simulink model "tpi2series"  (R2017b)
settings: Solver=VariableStepAuto  StartTime=0.0  StopTime=3  MaxStep=1e-4  RelTol=1e-3
values from neighbouring files (symbols this model uses):
  fdclinkcap = 100e-6    (= 0.0001)    [tpi2parallelrunner.m]    (also in tpi2seriesrunner.m = 0.01; tpireloadedrunner.m = 0.01)
  fdclinkres = 1e-6    (= 1e-06)    [tpi2parallelrunner.m]    (also in tpi2seriesrunner.m; tpireloadedrunner.m)
  fma = 0.9    [tpi2parallelrunner.m]    (also in tpi2seriesrunner.m; tpireloadedrunner.m)
  fswfreq = 20000    [tpi2parallelrunner.m]    (also in tpi2seriesrunner.m = 2050; tpireloadedrunner.m)
  Rin = 1    [tpi2parallelrunner.m]    (also in tpi2seriesrunner.m = 1e-16; tpireloadedrunner.m)
  sdclinkcap = 1e-2    (= 0.01)    [tpi2seriesrunner.m]    (also in tpireloadedrunner.m)
  sdclinkres = 1e-6    (= 1e-06)    [tpi2seriesrunner.m]    (also in tpireloadedrunner.m)
  sma = 0.9    [tpi2parallelrunner.m]    (also in tpi2seriesrunner.m; tpireloadedrunner.m)
  sswfreq = 20000    [tpi2parallelrunner.m]    (also in tpi2seriesrunner.m = 2050; tpireloadedrunner.m)
undefined symbols (not defined in the file or in its folder): fdcin, fdclink1cap
libraries: powerlib x22, simulink x6, powerlib_meascontrol x2
settings Model: Creator=Orhun  LastModifiedBy=Orhun

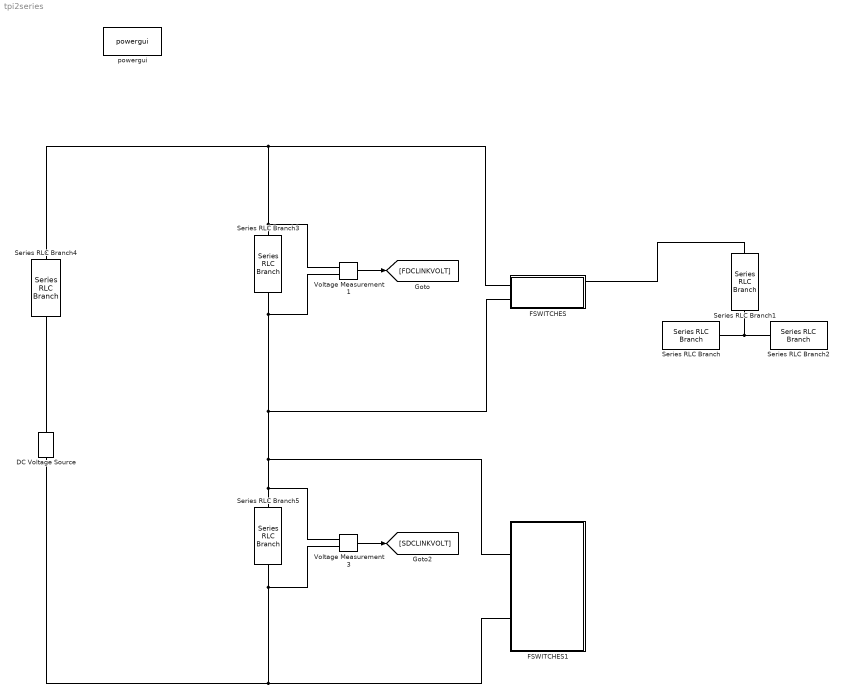
== system tpi2series ==
  DC Voltage Source : powerlib/Electrical Sources/DC Voltage Source  Amplitude=fdcin  Measurements=None
  FSWITCHES : Subsystem
  FSWITCHES1 : Subsystem
  Series RLC Branch : powerlib/Elements/Series RLC Branch  LConnTagsString=__new0  RConnTagsString=__new0  BranchType=RL  Resistance=5  Inductance=2e-3  SetiL0=off  InitialCurrent=0  Capacitance=0  Setx0=off  InitialVoltage=0  Measurements=None
  Series RLC Branch1 : powerlib/Elements/Series RLC Branch  LConnTagsString=__new0  RConnTagsString=__new0  BranchType=RL  Resistance=5  Inductance=2e-3  SetiL0=off  InitialCurrent=0  Capacitance=0  Setx0=off  InitialVoltage=0  Measurements=None
  Series RLC Branch2 : powerlib/Elements/Series RLC Branch  LConnTagsString=__new0  RConnTagsString=__new0  BranchType=RL  Resistance=5  Inductance=2e-3  SetiL0=off  InitialCurrent=0  Capacitance=0  Setx0=off  InitialVoltage=0  Measurements=None
  Series RLC Branch3 : powerlib/Elements/Series RLC Branch  LConnTagsString=__new0  RConnTagsString=__new0  BranchType=RC  Resistance=fdclinkres  Inductance=0  SetiL0=off  InitialCurrent=0  Capacitance=fdclinkcap  Setx0=off  InitialVoltage=0  Measurements=None
  Series RLC Branch4 : powerlib/Elements/Series RLC Branch  LConnTagsString=__new0  RConnTagsString=__new0  BranchType=R  Resistance=Rin  Inductance=0  SetiL0=off  InitialCurrent=0  Capacitance=fdclink1cap  Setx0=off  InitialVoltage=0  Measurements=None
  Series RLC Branch5 : powerlib/Elements/Series RLC Branch  LConnTagsString=__new0  RConnTagsString=__new0  BranchType=RC  Resistance=sdclinkres  Inductance=0  SetiL0=off  InitialCurrent=0  Capacitance=sdclinkcap  Setx0=off  InitialVoltage=0  Measurements=None
  Voltage Measurement1 : powerlib/Measurements/Voltage Measurement  PhasorSimulation=off  OutputType=Complex  PSBequivalent=0
  Voltage Measurement3 : powerlib/Measurements/Voltage Measurement  PhasorSimulation=off  OutputType=Complex  PSBequivalent=0
  powergui : powerlib/powergui  Priority=1  SimulationMode=Continuous  SampleTime=50e-6  frequency=60  Iterations=50  frequencyindice=0  Pbase=100e6  ErrMax=1e-4  UnitsV=kV  UnitsW=MW  buscounter=0  FunctionMessages=off  echomessages=off  EnableUseOfTLC=off  CurrentSourceSwitches=off  DisableSnubberDevices=off  DisableRonSwitches=off  DisableVfSwitches=off  DisplayEquations=off  SolverType=Tustin/Backward Euler (TBE)  Interpol=off  ExternalGateDelay=off  methode=off  Ts=100  x0status=blocks  SPID=on  SwTol=0  HookPort=off  RestoreLinks=warning  ResistiveCurrentMeasurement=off  Frange=[0:2:500]  Ylog=off  Xlog=on  ShowGrid=off  save=off  variable=ZData  structure=0  ZoomFFT=off  StartTime=0.0  cycles=1  DisplayStyle=1  fundamental=60  FreqAxis=off  MaxFrequency=1000  frequencyindicesteady=1  RmsSteady=1  display=off
  wires:
  Voltage Measurement1/1 -> [FDCLINKVOLT]
  Voltage Measurement3/1 -> [SDCLINKVOLT]
  connections:
  Series RLC Branch2/RConn1 -- Series RLC Branch1/LConn1 -- Series RLC Branch/LConn1
  Series RLC Branch3/LConn1 -- Series RLC Branch4/LConn1 -- FSWITCHES/LConn1 -- Voltage Measurement1/LConn1
  Voltage Measurement1/LConn2 -- FSWITCHES1/LConn1 -- Voltage Measurement3/LConn1 -- Series RLC Branch5/LConn1 -- FSWITCHES/LConn2 -- Series RLC Branch3/RConn1
  Series RLC Branch4/RConn1 -- DC Voltage Source/RConn1
  Voltage Measurement3/LConn2 -- DC Voltage Source/LConn1 -- FSWITCHES1/LConn2 -- Series RLC Branch5/RConn1
  FSWITCHES/RConn1 -- Series RLC Branch1/RConn1

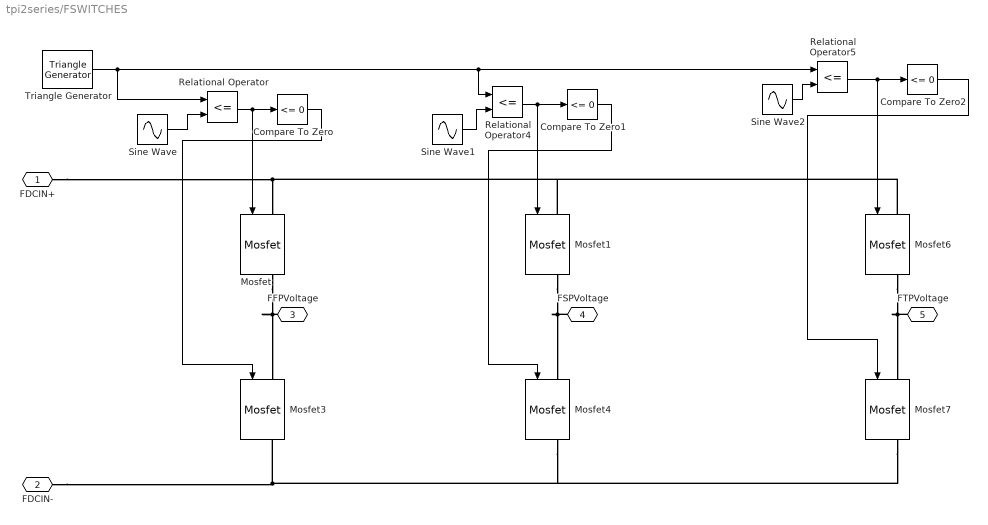
== system tpi2series/FSWITCHES ==
  Compare To Zero : simulink/Logic and Bit Operations/Compare To Zero  relop=<=  OutDataTypeStr=boolean
  Compare To Zero1 : simulink/Logic and Bit Operations/Compare To Zero  relop=<=  OutDataTypeStr=boolean
  Compare To Zero2 : simulink/Logic and Bit Operations/Compare To Zero  relop=<=  OutDataTypeStr=boolean
  Mosfet{,1,3..4,6..7} (6 alike) : powerlib/Power Electronics/Mosfet  Ron=2e-3  Lon=0  Rd=0.01  Vfd=0  IC=0  Rs=1e5  Cs=inf  Measurements=on
  Relational Operator : RelationalOperator  Operator=<=  OutDataTypeStr=boolean  RndMeth=Simplest
  Relational Operator4 : RelationalOperator  Operator=<=  OutDataTypeStr=boolean  RndMeth=Simplest
  Relational Operator5 : RelationalOperator  Operator=<=  OutDataTypeStr=boolean  RndMeth=Simplest
  Sine Wave : Sin  Amplitude=fma  Frequency=2*pi*fswfreq  SampleTime=0
  Sine Wave1 : Sin  Amplitude=fma  Frequency=2*pi*fswfreq  Phase=2*pi/3  SampleTime=0
  Sine Wave2 : Sin  Amplitude=fma  Frequency=2*pi*fswfreq  Phase=4*pi/3  SampleTime=0
  Triangle Generator : powerlib_meascontrol/Pulse & Signal Generators/Triangle Generator  Freq=fswfreq  Phase=90  Ts=0
  FDCIN+ : PMIOPort  Port=1  Side=Left
  FDCIN- : PMIOPort  Port=2  Side=Left
  FFPVoltage : PMIOPort  Port=3  Side=Right
  FSPVoltage : PMIOPort  Port=4  Side=Right
  FTPVoltage : PMIOPort  Port=5  Side=Right
  wires:
  Sine Wave/1 -> Relational Operator/2
  Triangle Generator/1 -> Relational Operator5/1, Relational Operator4/1, Relational Operator/1
  Relational Operator4/1 -> Mosfet1/1, Compare To Zero1/1
  Sine Wave2/1 -> Relational Operator5/2
  Sine Wave1/1 -> Relational Operator4/2
  Relational Operator/1 -> Compare To Zero/1, Mosfet/1
  Compare To Zero/1 -> Mosfet3/1
  Compare To Zero1/1 -> Mosfet4/1
  Compare To Zero2/1 -> Mosfet7/1
  Relational Operator5/1 -> Mosfet6/1, Compare To Zero2/1
  connections:
  Mosfet6/RConn1 -- FTPVoltage/RConn1 -- Mosfet7/LConn1
  Mosfet/RConn1 -- FFPVoltage/RConn1 -- Mosfet3/LConn1
  Mosfet1/RConn1 -- FSPVoltage/RConn1 -- Mosfet4/LConn1
  FDCIN+/RConn1 -- Mosfet6/LConn1 -- Mosfet1/LConn1 -- Mosfet/LConn1
  FDCIN-/RConn1 -- Mosfet4/RConn1 -- Mosfet7/RConn1 -- Mosfet3/RConn1

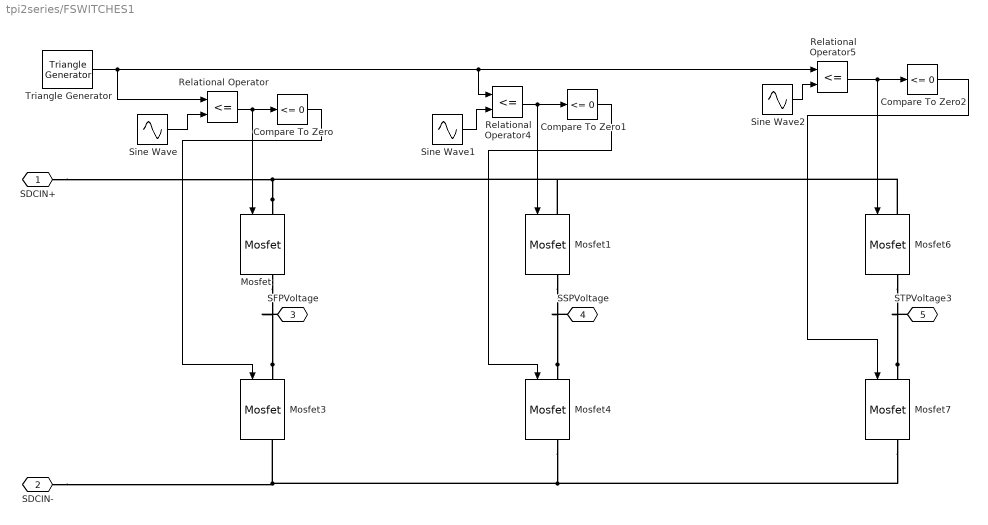
== system tpi2series/FSWITCHES1 ==
  Compare To Zero : simulink/Logic and Bit Operations/Compare To Zero  relop=<=  OutDataTypeStr=boolean
  Compare To Zero1 : simulink/Logic and Bit Operations/Compare To Zero  relop=<=  OutDataTypeStr=boolean
  Compare To Zero2 : simulink/Logic and Bit Operations/Compare To Zero  relop=<=  OutDataTypeStr=boolean
  Mosfet{,1,3..4,6..7} (6 alike) : powerlib/Power Electronics/Mosfet  Ron=2e-3  Lon=0  Rd=0.01  Vfd=0  IC=0  Rs=1e5  Cs=inf  Measurements=on
  Relational Operator : RelationalOperator  Operator=<=  OutDataTypeStr=boolean  RndMeth=Simplest
  Relational Operator4 : RelationalOperator  Operator=<=  OutDataTypeStr=boolean  RndMeth=Simplest
  Relational Operator5 : RelationalOperator  Operator=<=  OutDataTypeStr=boolean  RndMeth=Simplest
  Sine Wave : Sin  Amplitude=sma  Frequency=2*pi*sswfreq  SampleTime=0
  Sine Wave1 : Sin  Amplitude=sma  Frequency=2*pi*sswfreq  Phase=2*pi/3  SampleTime=0
  Sine Wave2 : Sin  Amplitude=fma  Frequency=2*pi*fswfreq  Phase=4*pi/3  SampleTime=0
  Triangle Generator : powerlib_meascontrol/Pulse & Signal Generators/Triangle Generator  Freq=sswfreq  Phase=90  Ts=0
  SDCIN+ : PMIOPort  Port=1  Side=Left
  SDCIN- : PMIOPort  Port=2  Side=Left
  SFPVoltage : PMIOPort  Port=3  Side=Right
  SSPVoltage : PMIOPort  Port=4  Side=Right
  STPVoltage3 : PMIOPort  Port=5  Side=Right
  wires:
  Sine Wave/1 -> Relational Operator/2
  Triangle Generator/1 -> Relational Operator5/1, Relational Operator4/1, Relational Operator/1
  Relational Operator4/1 -> Mosfet1/1, Compare To Zero1/1
  Sine Wave2/1 -> Relational Operator5/2
  Sine Wave1/1 -> Relational Operator4/2
  Relational Operator/1 -> Compare To Zero/1, Mosfet/1
  Compare To Zero/1 -> Mosfet3/1
  Compare To Zero1/1 -> Mosfet4/1
  Compare To Zero2/1 -> Mosfet7/1
  Relational Operator5/1 -> Mosfet6/1, Compare To Zero2/1
  connections:
  Mosfet7/LConn1 -- Mosfet6/RConn1 -- STPVoltage3/RConn1
  Mosfet3/LConn1 -- Mosfet/RConn1 -- SFPVoltage/RConn1
  Mosfet4/LConn1 -- Mosfet1/RConn1 -- SSPVoltage/RConn1
  Mosfet/LConn1 -- SDCIN+/RConn1 -- Mosfet6/LConn1 -- Mosfet1/LConn1
  Mosfet4/RConn1 -- Mosfet3/RConn1 -- SDCIN-/RConn1 -- Mosfet7/RConn1
